simulink library "TYPEA_GAS_MODAL_MASTER"  (Simulink 8.6)
settings: Solver=VariableStepAuto  StartTime=0.0  StopTime=10.0  RelTol=1e-3
libraries: cdsEpicsOut x11, cdsFiltCtrl x5, cdsEpicsIn x5, cdsFilt x5, cdsMuxMatrix x2, VIS_LIB x1
(part 1 of 2)
settings Model: Creator=controls  LastModifiedBy=controls

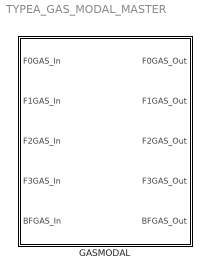
== system TYPEA_GAS_MODAL_MASTER ==
  GASMODAL : Subsystem

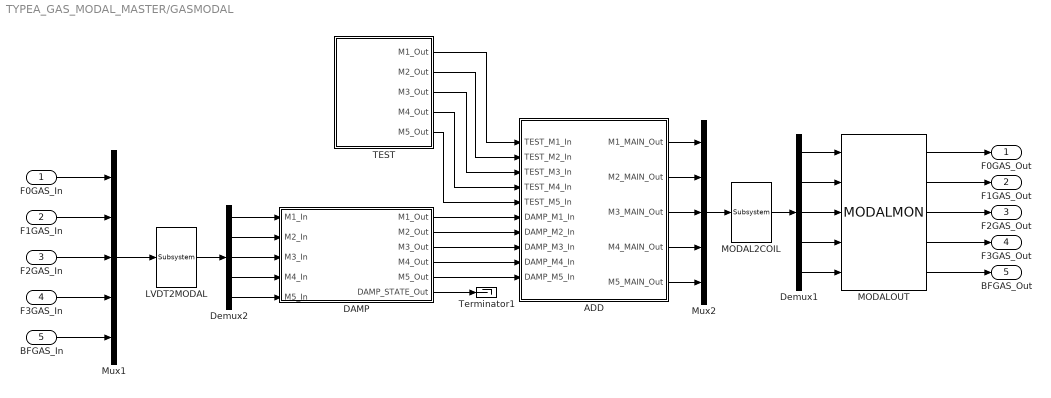
== system TYPEA_GAS_MODAL_MASTER/GASMODAL ==
  F0GAS_In : Inport
  F1GAS_In : Inport  Port=2
  F2GAS_In : Inport  Port=3
  F3GAS_In : Inport  Port=4
  BFGAS_In : Inport  Port=5
  ADD : Subsystem
  DAMP : Subsystem
  Demux1 : Demux  Outputs=5
  Demux2 : Demux  Outputs=5
  LVDT2MODAL : cdsMuxMatrix/Subsystem  Tag=cdsMuxMatrix  Description=Any size matrix. Inputs and outputs must be connected using Mux and Demux parts.
      settings: AttributesFormatString=%<Tag>
  MODAL2COIL : cdsMuxMatrix/Subsystem  Tag=cdsMuxMatrix  Description=Any size matrix. Inputs and outputs must be connected using Mux and Demux parts.
      settings: AttributesFormatString=%<Tag>
  MODALOUT : VIS_LIB/MODALMON
  Mux1 : Mux  Inputs=5
  Mux2 : Mux  Inputs=5
  TEST : Subsystem
  Terminator1 : Terminator
  F0GAS_Out : Outport
  F1GAS_Out : Outport  Port=2
  F2GAS_Out : Outport  Port=3
  F3GAS_Out : Outport  Port=4
  BFGAS_Out : Outport  Port=5
  wires:
  Mux1/1 -> LVDT2MODAL/1
  F3GAS_In/1 -> Mux1/4
  F0GAS_In/1 -> Mux1/1
  BFGAS_In/1 -> Mux1/5
  F2GAS_In/1 -> Mux1/3
  F1GAS_In/1 -> Mux1/2
  TEST/1(M1_Out) -> ADD/1(TEST_M1_In)
  TEST/2(M2_Out) -> ADD/2(TEST_M2_In)
  TEST/3(M3_Out) -> ADD/3(TEST_M3_In)
  TEST/4(M4_Out) -> ADD/4(TEST_M4_In)
  TEST/5(M5_Out) -> ADD/5(TEST_M5_In)
  LVDT2MODAL/1 -> Demux2/1
  Demux2/5 -> DAMP/5(M5_In)
  Demux2/1 -> DAMP/1(M1_In)
  Demux2/4 -> DAMP/4(M4_In)
  Demux2/3 -> DAMP/3(M3_In)
  Demux2/2 -> DAMP/2(M2_In)
  DAMP/6(DAMP_STATE_Out) -> Terminator1/1
  DAMP/3(M3_Out) -> ADD/8(DAMP_M3_In)
  DAMP/4(M4_Out) -> ADD/9(DAMP_M4_In)
  DAMP/2(M2_Out) -> ADD/7(DAMP_M2_In)
  DAMP/5(M5_Out) -> ADD/10(DAMP_M5_In)
  DAMP/1(M1_Out) -> ADD/6(DAMP_M1_In)
  ADD/3(M3_MAIN_Out) -> Mux2/3
  ADD/2(M2_MAIN_Out) -> Mux2/2
  ADD/1(M1_MAIN_Out) -> Mux2/1
  ADD/4(M4_MAIN_Out) -> Mux2/4
  ADD/5(M5_MAIN_Out) -> Mux2/5
  MODAL2COIL/1 -> Demux1/1
  Mux2/1 -> MODAL2COIL/1
  Demux1/1 -> MODALOUT/1
  Demux1/2 -> MODALOUT/2
  Demux1/3 -> MODALOUT/3
  Demux1/4 -> MODALOUT/4
  Demux1/5 -> MODALOUT/5
  MODALOUT/2 -> F1GAS_Out/1
  MODALOUT/1 -> F0GAS_Out/1
  MODALOUT/3 -> F2GAS_Out/1
  MODALOUT/4 -> F3GAS_Out/1
  MODALOUT/5 -> BFGAS_Out/1

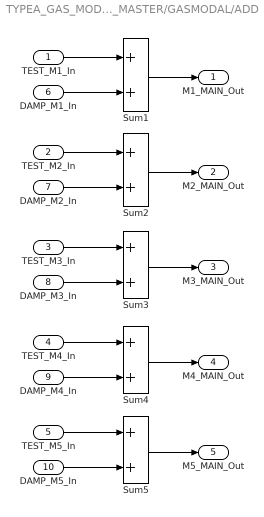
== system TYPEA_GAS_MODAL_MASTER/GASMODAL/ADD ==
  TEST_M1_In : Inport
  TEST_M2_In : Inport  Port=2
  TEST_M3_In : Inport  Port=3
  TEST_M4_In : Inport  Port=4
  TEST_M5_In : Inport  Port=5
  DAMP_M1_In : Inport  Port=6
  DAMP_M2_In : Inport  Port=7
  DAMP_M3_In : Inport  Port=8
  DAMP_M4_In : Inport  Port=9
  DAMP_M5_In : Inport  Port=10
  Sum{1..5} (5 alike) : Sum
  M1_MAIN_Out : Outport
  M2_MAIN_Out : Outport  Port=2
  M3_MAIN_Out : Outport  Port=3
  M4_MAIN_Out : Outport  Port=4
  M5_MAIN_Out : Outport  Port=5
  wires:
  Sum2/1 -> M2_MAIN_Out/1
  Sum1/1 -> M1_MAIN_Out/1
  Sum4/1 -> M4_MAIN_Out/1
  Sum3/1 -> M3_MAIN_Out/1
  DAMP_M1_In/1 -> Sum1/2
  TEST_M1_In/1 -> Sum1/1
  TEST_M2_In/1 -> Sum2/1
  DAMP_M2_In/1 -> Sum2/2
  TEST_M3_In/1 -> Sum3/1
  DAMP_M3_In/1 -> Sum3/2
  TEST_M4_In/1 -> Sum4/1
  DAMP_M4_In/1 -> Sum4/2
  Sum5/1 -> M5_MAIN_Out/1
  TEST_M5_In/1 -> Sum5/1
  DAMP_M5_In/1 -> Sum5/2

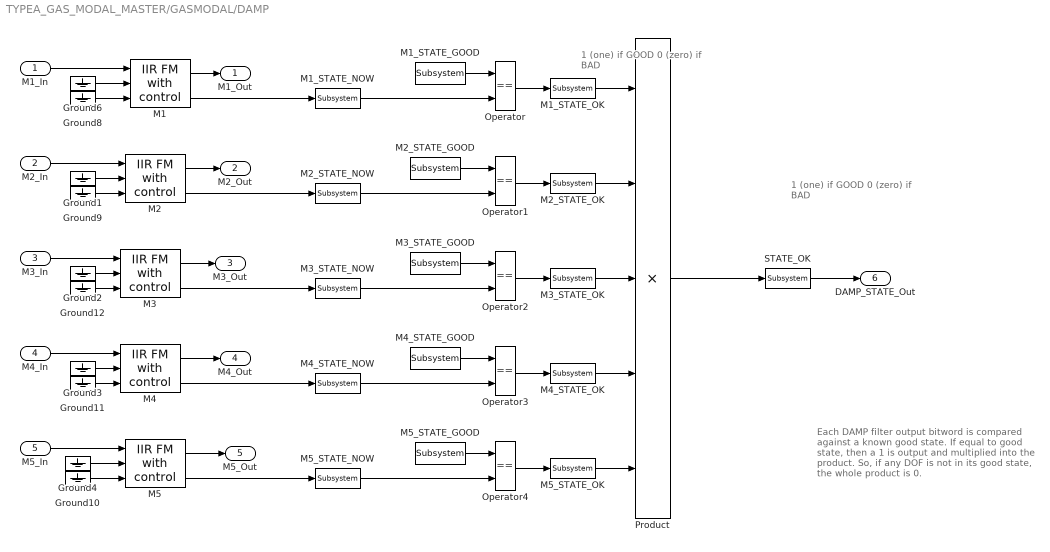
== system TYPEA_GAS_MODAL_MASTER/GASMODAL/DAMP ==
  note: 1 (one) if GOOD
      | 0 (zero) if BAD
  note: 1 (one) if GOOD
      | 0 (zero) if BAD
  note: Each DAMP filter output bitword is
      | compared against a known good state.
      | If equal to good state, then a 1 is output
      | and multiplied into the product. So, if any DOF
      | is not in its good state, the whole product is 0.
  M1_In : Inport
  M2_In : Inport  Port=2
  M3_In : Inport  Port=3
  M4_In : Inport  Port=4
  M5_In : Inport  Port=5
  Ground{1..4,6,8..12} (10 alike) : Ground
  M1 : cdsFiltCtrl/IIR FM with control  Tag=cdsFiltCtrl  Description=|
      | cdsFiltCntrl is the standard IIR filter module (exactly the same as cdsFilt) but with added control data output 'Ctrl'. Filter module digital signal output appears on the first output, which is called 'Val'. 'Ctrl' output has a bit pattern encoding the state of filter's on/off switches (FM1 through FM10). The bit values are:
      |                                                                                                                                                                                                                                                                                                                                       
      | module 	hex	dec                                                                                                                                                                                                                                                                                                                       
      | -----------------------                                                                                                                                                                                                                                                                                                               
      | FM1	0x20                    32                                                                                                                                                                                                                                                                                                        
      | FM2	0x80                     128                                                                                                                                                                                                                                                                                                      
      | FM3	0x200                   512                                                                                                                                                                                                                                                                                                       
      | FM4	0x800                   2048                                                                                                                                                                                                                                                                                                      
      | FM5	0x2000                 8192                                                                                                                                                                                                                                                                                                       
      | FM6	0x8000                 32768                                                                                                                                                                                                                                                                                                      
      | FM7	0x20000                131072                                                                                                                                                                                                                                                                                                     
      | FM8	0x80000                 524288                                                                                                                                                                                                                                                                                                    
      | FM9	0x200000               2097152                                                                                                                                                                                                                                                                                                    
      | FM10	0x800000               8388608                                                                                                                                                                                                                                                                                                   
      |                                                                                                                                                                                                                                                                                                                                       
      | This bit data can be used to drive some other switches or it can be output using a binary I/O module.
      settings: AttributesFormatString=%<Tag>
  M1_STATE_GOOD : cdsEpicsIn/Subsystem  Tag=cdsEpicsIn  Description=|
      | Purpose:                                                                              
      | Create an EPICS input channel connection to the FE realtime controls.                 
      |                                                                                       
      | Operation:                                                                            
      | Outputs value from an EPICS ai record. Value is floating point with a precision of 3..
      |                                                                                       
      | Usage:                                                                                
      | Name the part with the desired EPICS channel name.
      settings: AttributesFormatString=%<Tag>
  M1_STATE_NOW : cdsEpicsOut/Subsystem  Tag=cdsEpicsOutput  Description=|
      | Purpose:                                          
      | Output a FE signal to an EPICS channel.           
      |                                                   
      | Operation:                                        
      | Takes input value and passes it to EPICS record.  
      |                                                   
      | Usage:                                            
      | Name the part with the desired EPICS rrecord name.
      settings: AttributesFormatString=%<Tag>
  M1_STATE_OK : cdsEpicsOut/Subsystem  Tag=cdsEpicsOutput  Description=|
      | Purpose:                                          
      | Output a FE signal to an EPICS channel.           
      |                                                   
      | Operation:                                        
      | Takes input value and passes it to EPICS record.  
      |                                                   
      | Usage:                                            
      | Name the part with the desired EPICS rrecord name.
      settings: AttributesFormatString=%<Tag>
  M2 : cdsFiltCtrl/IIR FM with control  Tag=cdsFiltCtrl  Description=|
      | cdsFiltCntrl is the standard IIR filter module (exactly the same as cdsFilt) but with added control data output 'Ctrl'. Filter module digital signal output appears on the first output, which is called 'Val'. 'Ctrl' output has a bit pattern encoding the state of filter's on/off switches (FM1 through FM10). The bit values are:
      |                                                                                                                                                                                                                                                                                                                                       
      | module 	hex	dec                                                                                                                                                                                                                                                                                                                       
      | -----------------------                                                                                                                                                                                                                                                                                                               
      | FM1	0x20                    32                                                                                                                                                                                                                                                                                                        
      | FM2	0x80                     128                                                                                                                                                                                                                                                                                                      
      | FM3	0x200                   512                                                                                                                                                                                                                                                                                                       
      | FM4	0x800                   2048                                                                                                                                                                                                                                                                                                      
      | FM5	0x2000                 8192                                                                                                                                                                                                                                                                                                       
      | FM6	0x8000                 32768                                                                                                                                                                                                                                                                                                      
      | FM7	0x20000                131072                                                                                                                                                                                                                                                                                                     
      | FM8	0x80000                 524288                                                                                                                                                                                                                                                                                                    
      | FM9	0x200000               2097152                                                                                                                                                                                                                                                                                                    
      | FM10	0x800000               8388608                                                                                                                                                                                                                                                                                                   
      |                                                                                                                                                                                                                                                                                                                                       
      | This bit data can be used to drive some other switches or it can be output using a binary I/O module.
      settings: AttributesFormatString=%<Tag>
  M2_STATE_GOOD : cdsEpicsIn/Subsystem  Tag=cdsEpicsIn  Description=|
      | Purpose:                                                                              
      | Create an EPICS input channel connection to the FE realtime controls.                 
      |                                                                                       
      | Operation:                                                                            
      | Outputs value from an EPICS ai record. Value is floating point with a precision of 3..
      |                                                                                       
      | Usage:                                                                                
      | Name the part with the desired EPICS channel name.
      settings: AttributesFormatString=%<Tag>
  M2_STATE_NOW : cdsEpicsOut/Subsystem  Tag=cdsEpicsOutput  Description=|
      | Purpose:                                          
      | Output a FE signal to an EPICS channel.           
      |                                                   
      | Operation:                                        
      | Takes input value and passes it to EPICS record.  
      |                                                   
      | Usage:                                            
      | Name the part with the desired EPICS rrecord name.
      settings: AttributesFormatString=%<Tag>
  M2_STATE_OK : cdsEpicsOut/Subsystem  Tag=cdsEpicsOutput  Description=|
      | Purpose:                                          
      | Output a FE signal to an EPICS channel.           
      |                                                   
      | Operation:                                        
      | Takes input value and passes it to EPICS record.  
      |                                                   
      | Usage:                                            
      | Name the part with the desired EPICS rrecord name.
      settings: AttributesFormatString=%<Tag>
  M3 : cdsFiltCtrl/IIR FM with control  Tag=cdsFiltCtrl  Description=|
      | cdsFiltCntrl is the standard IIR filter module (exactly the same as cdsFilt) but with added control data output 'Ctrl'. Filter module digital signal output appears on the first output, which is called 'Val'. 'Ctrl' output has a bit pattern encoding the state of filter's on/off switches (FM1 through FM10). The bit values are:
      |                                                                                                                                                                                                                                                                                                                                       
      | module 	hex	dec                                                                                                                                                                                                                                                                                                                       
      | -----------------------                                                                                                                                                                                                                                                                                                               
      | FM1	0x20                    32                                                                                                                                                                                                                                                                                                        
      | FM2	0x80                     128                                                                                                                                                                                                                                                                                                      
      | FM3	0x200                   512                                                                                                                                                                                                                                                                                                       
      | FM4	0x800                   2048                                                                                                                                                                                                                                                                                                      
      | FM5	0x2000                 8192                                                                                                                                                                                                                                                                                                       
      | FM6	0x8000                 32768                                                                                                                                                                                                                                                                                                      
      | FM7	0x20000                131072                                                                                                                                                                                                                                                                                                     
      | FM8	0x80000                 524288                                                                                                                                                                                                                                                                                                    
      | FM9	0x200000               2097152                                                                                                                                                                                                                                                                                                    
      | FM10	0x800000               8388608                                                                                                                                                                                                                                                                                                   
      |                                                                                                                                                                                                                                                                                                                                       
      | This bit data can be used to drive some other switches or it can be output using a binary I/O module.
      settings: AttributesFormatString=%<Tag>
  M3_STATE_GOOD : cdsEpicsIn/Subsystem  Tag=cdsEpicsIn  Description=|
      | Purpose:                                                                              
      | Create an EPICS input channel connection to the FE realtime controls.                 
      |                                                                                       
      | Operation:                                                                            
      | Outputs value from an EPICS ai record. Value is floating point with a precision of 3..
      |                                                                                       
      | Usage:                                                                                
      | Name the part with the desired EPICS channel name.
      settings: AttributesFormatString=%<Tag>
  M3_STATE_NOW : cdsEpicsOut/Subsystem  Tag=cdsEpicsOutput  Description=|
      | Purpose:                                          
      | Output a FE signal to an EPICS channel.           
      |                                                   
      | Operation:                                        
      | Takes input value and passes it to EPICS record.  
      |                                                   
      | Usage:                                            
      | Name the part with the desired EPICS rrecord name.
      settings: AttributesFormatString=%<Tag>
  M3_STATE_OK : cdsEpicsOut/Subsystem  Tag=cdsEpicsOutput  Description=|
      | Purpose:                                          
      | Output a FE signal to an EPICS channel.           
      |                                                   
      | Operation:                                        
      | Takes input value and passes it to EPICS record.  
      |                                                   
      | Usage:                                            
      | Name the part with the desired EPICS rrecord name.
      settings: AttributesFormatString=%<Tag>
  M4 : cdsFiltCtrl/IIR FM with control  Tag=cdsFiltCtrl  Description=|
      | cdsFiltCntrl is the standard IIR filter module (exactly the same as cdsFilt) but with added control data output 'Ctrl'. Filter module digital signal output appears on the first output, which is called 'Val'. 'Ctrl' output has a bit pattern encoding the state of filter's on/off switches (FM1 through FM10). The bit values are:
      |                                                                                                                                                                                                                                                                                                                                       
      | module 	hex	dec                                                                                                                                                                                                                                                                                                                       
      | -----------------------                                                                                                                                                                                                                                                                                                               
      | FM1	0x20                    32                                                                                                                                                                                                                                                                                                        
      | FM2	0x80                     128                                                                                                                                                                                                                                                                                                      
      | FM3	0x200                   512                                                                                                                                                                                                                                                                                                       
      | FM4	0x800                   2048                                                                                                                                                                                                                                                                                                      
      | FM5	0x2000                 8192                                                                                                                                                                                                                                                                                                       
      | FM6	0x8000                 32768                                                                                                                                                                                                                                                                                                      
      | FM7	0x20000                131072                                                                                                                                                                                                                                                                                                     
      | FM8	0x80000                 524288                                                                                                                                                                                                                                                                                                    
      | FM9	0x200000               2097152                                                                                                                                                                                                                                                                                                    
      | FM10	0x800000               8388608                                                                                                                                                                                                                                                                                                   
      |                                                                                                                                                                                                                                                                                                                                       
      | This bit data can be used to drive some other switches or it can be output using a binary I/O module.
      settings: AttributesFormatString=%<Tag>
  M4_STATE_GOOD : cdsEpicsIn/Subsystem  Tag=cdsEpicsIn  Description=|
      | Purpose:                                                                              
      | Create an EPICS input channel connection to the FE realtime controls.                 
      |                                                                                       
      | Operation:                                                                            
      | Outputs value from an EPICS ai record. Value is floating point with a precision of 3..
      |                                                                                       
      | Usage:                                                                                
      | Name the part with the desired EPICS channel name.
      settings: AttributesFormatString=%<Tag>
  M4_STATE_NOW : cdsEpicsOut/Subsystem  Tag=cdsEpicsOutput  Description=|
      | Purpose:                                          
      | Output a FE signal to an EPICS channel.           
      |                                                   
      | Operation:                                        
      | Takes input value and passes it to EPICS record.  
      |                                                   
      | Usage:                                            
      | Name the part with the desired EPICS rrecord name.
      settings: AttributesFormatString=%<Tag>
  M4_STATE_OK : cdsEpicsOut/Subsystem  Tag=cdsEpicsOutput  Description=|
      | Purpose:                                          
      | Output a FE signal to an EPICS channel.           
      |                                                   
      | Operation:                                        
      | Takes input value and passes it to EPICS record.  
      |                                                   
      | Usage:                                            
      | Name the part with the desired EPICS rrecord name.
      settings: AttributesFormatString=%<Tag>
  M5 : cdsFiltCtrl/IIR FM with control  Tag=cdsFiltCtrl  Description=|
      | cdsFiltCntrl is the standard IIR filter module (exactly the same as cdsFilt) but with added control data output 'Ctrl'. Filter module digital signal output appears on the first output, which is called 'Val'. 'Ctrl' output has a bit pattern encoding the state of filter's on/off switches (FM1 through FM10). The bit values are:
      |                                                                                                                                                                                                                                                                                                                                       
      | module 	hex	dec                                                                                                                                                                                                                                                                                                                       
      | -----------------------                                                                                                                                                                                                                                                                                                               
      | FM1	0x20                    32                                                                                                                                                                                                                                                                                                        
      | FM2	0x80                     128                                                                                                                                                                                                                                                                                                      
      | FM3	0x200                   512                                                                                                                                                                                                                                                                                                       
      | FM4	0x800                   2048                                                                                                                                                                                                                                                                                                      
      | FM5	0x2000                 8192                                                                                                                                                                                                                                                                                                       
      | FM6	0x8000                 32768                                                                                                                                                                                                                                                                                                      
      | FM7	0x20000                131072                                                                                                                                                                                                                                                                                                     
      | FM8	0x80000                 524288                                                                                                                                                                                                                                                                                                    
      | FM9	0x200000               2097152                                                                                                                                                                                                                                                                                                    
      | FM10	0x800000               8388608                                                                                                                                                                                                                                                                                                   
      |                                                                                                                                                                                                                                                                                                                                       
      | This bit data can be used to drive some other switches or it can be output using a binary I/O module.
      settings: AttributesFormatString=%<Tag>
  M5_STATE_GOOD : cdsEpicsIn/Subsystem  Tag=cdsEpicsIn  Description=|
      | Purpose:                                                                              
      | Create an EPICS input channel connection to the FE realtime controls.                 
      |                                                                                       
      | Operation:                                                                            
      | Outputs value from an EPICS ai record. Value is floating point with a precision of 3..
      |                                                                                       
      | Usage:                                                                                
      | Name the part with the desired EPICS channel name.
      settings: AttributesFormatString=%<Tag>
  M5_STATE_NOW : cdsEpicsOut/Subsystem  Tag=cdsEpicsOutput  Description=|
      | Purpose:                                          
      | Output a FE signal to an EPICS channel.           
      |                                                   
      | Operation:                                        
      | Takes input value and passes it to EPICS record.  
      |                                                   
      | Usage:                                            
      | Name the part with the desired EPICS rrecord name.
      settings: AttributesFormatString=%<Tag>
  M5_STATE_OK : cdsEpicsOut/Subsystem  Tag=cdsEpicsOutput  Description=|
      | Purpose:                                          
      | Output a FE signal to an EPICS channel.           
      |                                                   
      | Operation:                                        
      | Takes input value and passes it to EPICS record.  
      |                                                   
      | Usage:                                            
      | Name the part with the desired EPICS rrecord name.
      settings: AttributesFormatString=%<Tag>
  Operator{,1..4} (5 alike) : RelationalOperator  Operator===  OutDataTypeStr=boolean
  Product : Product  Inputs=5  RndMeth=Zero
  STATE_OK : cdsEpicsOut/Subsystem  Tag=cdsEpicsOutput  Description=|
      | Purpose:                                          
      | Output a FE signal to an EPICS channel.           
      |                                                   
      | Operation:                                        
      | Takes input value and passes it to EPICS record.  
      |                                                   
      | Usage:                                            
      | Name the part with the desired EPICS rrecord name.
      settings: AttributesFormatString=%<Tag>
  M1_Out : Outport
  M2_Out : Outport  Port=2
  M3_Out : Outport  Port=3
  M4_Out : Outport  Port=4
  M5_Out : Outport  Port=5
  DAMP_STATE_Out : Outport  Port=6
  wires:
  Ground12/1 -> M3/3
  Ground11/1 -> M4/3
  Ground10/1 -> M5/3
  Ground9/1 -> M2/3
  Ground8/1 -> M1/3
  STATE_OK/1 -> DAMP_STATE_Out/1
  M5_STATE_NOW/1 -> Operator4/2
  M4_STATE_NOW/1 -> Operator3/2
  M3_STATE_NOW/1 -> Operator2/2
  M2_STATE_NOW/1 -> Operator1/2
  M1_STATE_NOW/1 -> Operator/2
  M5_STATE_OK/1 -> Product/5
  M4_STATE_OK/1 -> Product/4
  M3_STATE_OK/1 -> Product/3
  M2_STATE_OK/1 -> Product/2
  M1_STATE_OK/1 -> Product/1
  Operator4/1 -> M5_STATE_OK/1
  Operator3/1 -> M4_STATE_OK/1
  Operator2/1 -> M3_STATE_OK/1
  Operator1/1 -> M2_STATE_OK/1
  Operator/1 -> M1_STATE_OK/1
  Product/1 -> STATE_OK/1
  M5/2 -> M5_STATE_NOW/1
  M5_STATE_GOOD/1 -> Operator4/1
  M4/2 -> M4_STATE_NOW/1
  M4_STATE_GOOD/1 -> Operator3/1
  M3/2 -> M3_STATE_NOW/1
  M3_STATE_GOOD/1 -> Operator2/1
  M2/2 -> M2_STATE_NOW/1
  M2_STATE_GOOD/1 -> Operator1/1
  M1/2 -> M1_STATE_NOW/1
  M1_STATE_GOOD/1 -> Operator/1
  M2_In/1 -> M2/1
  M3_In/1 -> M3/1
  M4_In/1 -> M4/1
  M5_In/1 -> M5/1
  M2/1 -> M2_Out/1
  M3/1 -> M3_Out/1
  M1/1 -> M1_Out/1
  M1_In/1 -> M1/1
  Ground4/1 -> M5/2
  Ground3/1 -> M4/2
  Ground2/1 -> M3/2
  Ground1/1 -> M2/2
  Ground6/1 -> M1/2
  M5/1 -> M5_Out/1
  M4/1 -> M4_Out/1
